simulink model "c28069_SCIledBpwm_T"  (R2018b)
settings: Solver=ode4  StartTime=0.0  StopTime=0.5  FixedStep=Ts  RelTol=1e-3
InitFcn:
  | Ts=1e-4
undefined symbols (not defined in the file): serial
libraries: instrumentlib x4
settings Model: Creator=matti  LastModifiedBy=matti
settings HardwareCC: ProdBitPerPointer=32  ProdBitPerSizeT=32  ProdBitPerPtrDiffT=32  ProdWordSize=32  ProdHWDeviceType=Intel->x86-32 (Windows32)
settings SFSimCC: SimUseLocalCustomCode=off
settings RTWCC: RTWUseLocalCustomCode=off
settings CodeAppCC: StateflowObjectComments=on
settings SimscapeCC: SimscapeNormalizeSystem=off

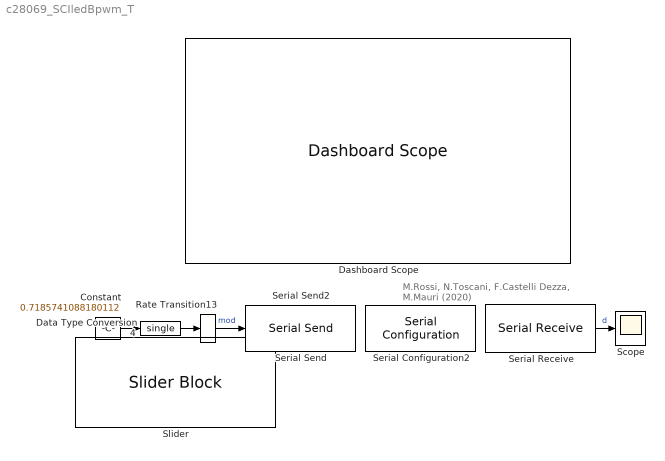
== system c28069_SCIledBpwm_T ==
  note: M.Rossi, N.Toscani, F.Castelli Dezza, M.Mauri (2020)
  Constant : Constant  Value=0.7185741088180112  SampleTime=Ts
  Dashboard Scope : DashboardScope  WebBlockId=52  TimeSpan=20  Ymin=-0.10000000000000001  Ymax=1.1000000000000001
  Data Type Conversion4 : DataTypeConversion  OutDataTypeStr=single
  Rate Transition13 : RateTransition  Integrity=off  OutPortSampleTime=0.01
  Scope : Scope
  Serial Configuration2 : instrumentlib/Serial Configuration  Priority=-200000  ComPortMenu=<Please select a port...>  ComPort=COM14  ObjConstructor=serial('COM14');  BaudRate=115200  DataBits=8  Parity=none  StopBits=1  FlowControl=none  Timeout=10  ByteOrder=LittleEndian
  Serial Receive : instrumentlib/Serial Receive  ComPortMenu=<Please select a port...>  ComPort=COM14  ObjConstructor=serial('COM14');  Terminator=<none>  DataSize="[1  1]"  DataType=single  EnableBlockingMode=on  ActionDataUnavailable=Output last received value  CustomValue=0  SampleTime=0.01
  Serial Send : instrumentlib/Serial Send  ComPortMenu=<Please select a port...>  ComPort=COM14  ObjConstructor=serial('COM14');  Terminator=<none>  EnableBlockingMode=on
  Serial Send2 : instrumentlib/Serial Send  ComPortMenu=<Please select a port...>  ComPort=COM14  ObjConstructor=serial('COM14');  Terminator=<none>  EnableBlockingMode=on
  Slider : SliderBlock  WebBlockId=120  LabelPosition=Hide  ScaleMax=1  TickInterval=0.5
  wires:
  Constant/1 -> Data Type Conversion4/1
  Rate Transition13/1 -> Serial Send/1  "mod"
  Data Type Conversion4/1 -> Rate Transition13/1
  Serial Receive/1 -> Scope/1  "d"
